simulink model "main"  (R2024a)
settings: Solver=FixedStepDiscrete  StartTime=0.0  StopTime=5  RelTol=1e-3
PreLoadFcn:
  | RTWConfigurationCB('preloadfcn', bdroot);
model workspace (MAT data in the model file):
  fault_count = 0
undefined symbols (not defined in the file or in its folder): Call, Function
libraries: canmsglib x15, c280xlib x13, c2837xDlib x9, c2802xlib x8, simulink x4, slpidlib x1
(part 2 of 2)

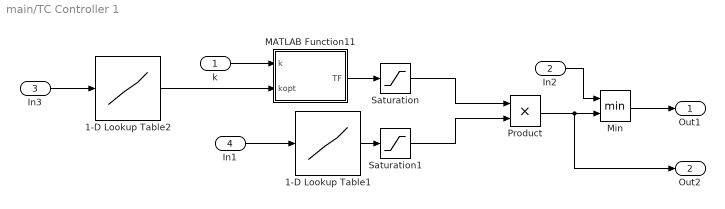
== system main/TC Controller 1 ==
  k : Inport
  In2 : Inport  Port=2
  In3 : Inport  Port=3
  In1 : Inport  Port=4
  1-D Lookup Table1 : Lookup_n-D  NumberOfTableDimensions=1  BreakpointsForDimension1=[1;10]  Table=[0;166]  ExtrapMethod=Clip  InternalRulePriority=Speed  RndMeth=Simplest
  1-D Lookup Table2 : Lookup_n-D  NumberOfTableDimensions=1  BreakpointsForDimension1=[1;10]  Table=[0.03;0.21]  ExtrapMethod=Clip  InternalRulePriority=Speed  RndMeth=Simplest
  MATLAB Function11 : MATLAB Function  TreatAsAtomicUnit=on
  Min : MinMax  Inputs=2
  Product : Product
  Saturation : Saturate  UpperLimit=1  LowerLimit=.1
  Saturation1 : Saturate  UpperLimit=166  LowerLimit=0
  Out1 : Outport
  Out2 : Outport  Port=2
  wires:
  1-D Lookup Table2/1 -> MATLAB Function11/2(kopt)
  MATLAB Function11/1(TF) -> Saturation/1
  Product/1 -> Out2/1, Min/2
  In1/1 -> 1-D Lookup Table1/1
  In2/1 -> Min/1
  1-D Lookup Table1/1 -> Saturation1/1
  Saturation1/1 -> Product/2
  Saturation/1 -> Product/1
  Min/1 -> Out1/1
  k/1 -> MATLAB Function11/1(k)
  In3/1 -> 1-D Lookup Table2/1

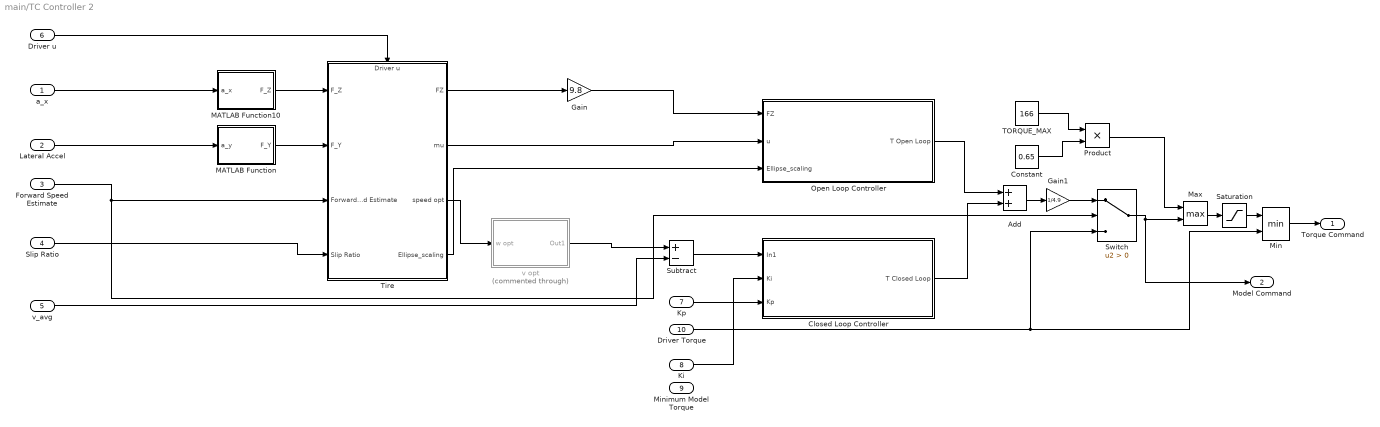
== system main/TC Controller 2 ==
  a_x : Inport
  Lateral Accel : Inport  Port=2
  Forward Speed Estimate : Inport  Port=3
  Slip Ratio : Inport  Port=4
  v_avg : Inport  Port=5
  Driver u : Inport  Port=6
  Kp : Inport  Port=7
  Ki : Inport  Port=8
  Minimum Model Torque : Inport  Port=9
  Driver Torque : Inport  Port=10
  Add : Sum
  Closed Loop Controller : Subsystem
  Constant : Constant  Value=0.65
  Gain : Gain  Gain=9.8
  Gain1 : Gain  Gain=1/4.9
  MATLAB Function : MATLAB Function  TreatAsAtomicUnit=on
  MATLAB Function10 : MATLAB Function  TreatAsAtomicUnit=on
  Max : MinMax  Function=max  Inputs=2
  Min : MinMax  Inputs=2
  Open Loop Controller : Subsystem
  Product : Product
  Saturation : Saturate  UpperLimit=166  LowerLimit=0
  Subtract : Sum  Inputs=+-
  Switch : Switch  Criteria=u2 > Threshold  SaturateOnIntegerOverflow=off  InputSameDT=off
  TORQUE_MAX : Constant  Value=166
  Tire : Subsystem
      settings: PortSchema="{\"entries\":[{\"content\":{\"sides\":[{\"content\":{\"connectorIds\":[\"In1\",\"In2\",\"In3\",\"In4\"]},\"type\":\"ConnectorPlacement.EquallySpacedRectSide\",\"uuid\":\"4156dcb8-571a-4ee4-a7f1-7560a1681aa7\"},{\"content\":{\"connectorIds\":[\"Out1\",\"Out2\",\"Out3\",\"Out4\"],\"side\":\"RIGHT\"},\"type\":\"ConnectorPlacement.EquallySpacedRectSide\",\"uuid\":\"73638d28-b906-4671-b83f-ad6b48e8d393\"},{\"content\":{\"connectorIds\":[\"In5\"],\"side\":\"TOP\"},\"type\":\"ConnectorPlacement.EquallySpacedRectSide\",\"uuid\":\"2e0ca522-3e79-4dd0-9128-59b05a2bd3de\"}]},\"type\":\"ConnectorPlacement.EquallySpacedConnector\",\"uuid\":\"62676716-b41d-4cd9-a12c-b09e0afde3e3\"}],\"packageUris\":[\"http://schema.mathworks.com/mf0/Connector/R2020b\"],\"version\":\"1.0\"}"
  v opt : Subsystem  Commented=through
  Torque Command : Outport
  Model Command : Outport  Port=2
  wires:
  Gain1/1 -> Switch/1
  Tire/2(mu) -> Open Loop Controller/2(u)
  a_x/1 -> MATLAB Function10/1(a_x)
  MATLAB Function10/1(F_Z) -> Tire/1(F_Z)
  Open Loop Controller/1(T Open Loop) -> Add/1
  Closed Loop Controller/1(T Closed Loop) -> Add/2
  v opt/1(Out1) -> Subtract/1
  Tire/3(speed opt) -> v opt/1(w opt)
  Subtract/1 -> Closed Loop Controller/1(In1)
  Add/1 -> Gain1/1
  Tire/1(FZ) -> Gain/1
  Driver u/1 -> Tire/5(Driver u)
  v_avg/1 -> Subtract/2
  Slip Ratio/1 -> Tire/4(Slip Ratio)
  Kp/1 -> Closed Loop Controller/3(Kp)
  Saturation/1 -> Min/1
  Gain/1 -> Open Loop Controller/1(FZ)
  Forward Speed Estimate/1 -> Switch/2, Tire/3(Forward Speed Estimate)
  Switch/1 -> Max/2, Model Command/1
  Driver Torque/1 -> Min/2, Switch/3
  Min/1 -> Torque Command/1
  Ki/1 -> Closed Loop Controller/2(Ki)
  Max/1 -> Saturation/1
  TORQUE_MAX/1 -> Product/1
  Constant/1 -> Product/2
  Product/1 -> Max/1
  MATLAB Function/1(F_Y) -> Tire/2(F_Y)
  Lateral Accel/1 -> MATLAB Function/1(a_y)
  Tire/4(Ellipse_scaling) -> Open Loop Controller/3(Ellipse_scaling)

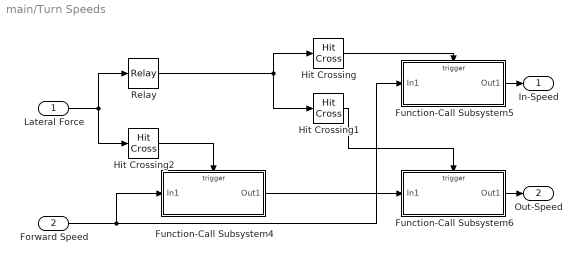
== system main/Turn Speeds ==
  Lateral Force : Inport
  Forward Speed : Inport  Port=2
  Function-Call Subsystem4 : Subsystem  TreatAsAtomicUnit=on
  Function-Call Subsystem5 : Subsystem  TreatAsAtomicUnit=on
  Function-Call Subsystem6 : Subsystem  TreatAsAtomicUnit=on
  Hit Crossing : HitCross  HitCrossingOffset=0.5  HitCrossingDirection=rising  HitCrossingOutputType=Function-Call
  Hit Crossing1 : HitCross  HitCrossingOffset=0.5  HitCrossingDirection=falling  HitCrossingOutputType=Function-Call
  Hit Crossing2 : HitCross  HitCrossingOffset=1  HitCrossingOutputType=Function-Call
  Relay : Relay  OnSwitchValue=1  OffSwitchValue=0.5
  In-Speed : Outport
  Out-Speed : Outport  Port=2
  wires:
  Forward Speed/1 -> Function-Call Subsystem4/1(In1), Function-Call Subsystem5/1(In1)
  Hit Crossing2/1 -> Function-Call Subsystem4/Trigger
  Function-Call Subsystem4/1(Out1) -> Function-Call Subsystem6/1(In1)
  Relay/1 -> Hit Crossing1/1, Hit Crossing/1
  Hit Crossing1/1 -> Function-Call Subsystem6/Trigger
  Hit Crossing/1 -> Function-Call Subsystem5/Trigger
  Function-Call Subsystem5/1(Out1) -> In-Speed/1
  Lateral Force/1 -> Relay/1, Hit Crossing2/1
  Function-Call Subsystem6/1(Out1) -> Out-Speed/1

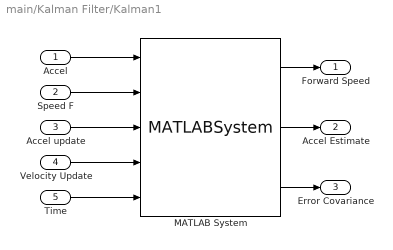
== system main/Kalman Filter/Kalman1 ==
  Accel : Inport
  Speed F : Inport  Port=2
  Accel update : Inport  Port=3
  Velocity Update : Inport  Port=4
  Time : Inport  Port=5
  MATLAB System : MATLABSystem  System=Kalman_Filter_Mod  qgain=1  SimulateUsing=Code generation
      mask Type: Kalman_Filter_Mod
      mask Display:
      | disp('Kalman_Filter_Mod');
      | port_label('input',1,'a');
      | port_label('input',2,'v_f');
      | port_label('input',3,'n_a');
      | port_label('input',4,'n_v');
      | port_label('input',5,'t_new');
      | port_label('output',1,'v');
      | port_label('output',2,'a');
      | port_label('output',3,'cov_v');
  Forward Speed : Outport
  Accel Estimate : Outport  Port=2
  Error Covariance : Outport  Port=3
  wires:
  Speed F/1 -> MATLAB System/2
  Accel/1 -> MATLAB System/1
  MATLAB System/1 -> Forward Speed/1
  Accel update/1 -> MATLAB System/3
  Velocity Update/1 -> MATLAB System/4
  Time/1 -> MATLAB System/5
  MATLAB System/2 -> Accel Estimate/1
  MATLAB System/3 -> Error Covariance/1

== system main/Kalman Filter/Sensor Driver 1 ==
  In1 : Inport
  Circumference : Gain  Gain=2*pi*0.203
  Gain : Gain  Gain=3.6
  Inverse Teeth : Gain  Gain=1/21
  " " : Outport
  wires:
  In1/1 -> Gain/1
  Gain/1 -> Circumference/1
  Circumference/1 -> Inverse Teeth/1
  Inverse Teeth/1 -> " "/1

== system main/Kalman Filter/Sensor Driver 2 ==
  In1 : Inport
  Circumference : Gain  Gain=2*pi*0.203
  Gain : Gain  Gain=3.6
  Inverse Teeth : Gain  Gain=1/21
  " " : Outport
  wires:
  Circumference/1 -> Inverse Teeth/1
  Inverse Teeth/1 -> " "/1
  In1/1 -> Gain/1
  Gain/1 -> Circumference/1

== system main/Kalman Filter/Sensor Driver 3 ==
  In1 : Inport
  Circumference : Gain  Gain=2*pi*0.203
  Gain : Gain  Gain=3.6
  Inverse Teeth : Gain  Gain=1/21
  RL : Outport
  wires:
  Circumference/1 -> Inverse Teeth/1
  Inverse Teeth/1 -> RL/1
  In1/1 -> Gain/1
  Gain/1 -> Circumference/1

== system main/Kalman Filter/Sensor Driver 4 ==
  In1 : Inport
  Circumference : Gain  Gain=2*pi*0.203
  Gain : Gain  Gain=3.6
  Inverse Teeth : Gain  Gain=1/21
  RR : Outport
  wires:
  Circumference/1 -> Inverse Teeth/1
  Inverse Teeth/1 -> RR/1
  In1/1 -> Gain/1
  Gain/1 -> Circumference/1

== system main/Kalman Filter/Slip Ratio Calculation1 ==
  RR : Inport
  Forward Speed : Inport  Port=2
  MATLAB Function : MATLAB Function  TreatAsAtomicUnit=on
  Slip Ratio : Outport
  wires:
  Forward Speed/1 -> MATLAB Function/1(fwd_speed)
  RR/1 -> MATLAB Function/2(v_rear)
  MATLAB Function/1(y) -> Slip Ratio/1

== system main/Power Limiting/Moving Average ==
  In1 : Inport
  Product1 : Product  Inputs=*/
  Saturation : Saturate  UpperLimit=inf  LowerLimit=1
  Sum of Elements : Sum  Inputs=+
  Tapped Delay : simulink/Discrete/Tapped Delay  vinit=0.0  samptime=-1  NumDelays=10  DelayOrder=Oldest  includeCurrent=on
  Width : Width
  Out1 : Outport
  wires:
  Tapped Delay/1 -> Width/1, Sum of Elements/1
  Sum of Elements/1 -> Product1/1
  Product1/1 -> Out1/1
  In1/1 -> Tapped Delay/1
  Width/1 -> Saturation/1
  Saturation/1 -> Product1/2

== system main/TC Controller 2/Closed Loop Controller ==
  In1 : Inport
  Ki : Inport  Port=2
  Kp : Inport  Port=3
  Constant : Constant  Value=2
  Divide : Product  Inputs=*/
  PID Controller : slpidlib/PID Controller  Controller=PI  Form=Parallel  TimeDomain=Discrete-time  UseExternalTs=off  SampleTime=-1  IntegratorMethod=Forward Euler  FilterMethod=Forward Euler  ControllerParametersSource=external  P=100  I=10  UseKiTs=off  D=0  UseExternalDerivativeSource=off  N=100  UseFilter=on  TunerSelectOption=Transfer Function Based (PID Tuner App)  InitialConditionSource=internal  InitialConditionForIntegrator=0  InitialConditionForFilter=0  DifferentiatorICPrevScaledInput=0  ExternalReset=none  TrackingMode=off  Kt=1  LimitOutput=on  SatLimitsSource=internal  UpperSaturationLimit=166  LowerSaturationLimit=0  LinearizeAsGain=on  AntiWindupMode=clamping  Kb=1  LimitIntegrator=on  UpperIntegratorSaturationLimit=166  LowerIntegratorSaturationLimit=0  POutMin=[]  POutMax=[]  IOutMin=[]  IOutMax=[]  DOutMin=[]  DOutMax=[]  NOutMin=[]  NOutMax=[]  SumOutMin=[]  SumOutMax=[]  SaturationOutMin=[]  SaturationOutMax=[]  PParamMin=[]  PParamMax=[]  IParamMin=[]  IParamMax=[]  DParamMin=[]  DParamMax=[]  NParamMin=[]  NParamMax=[]  KbParamMin=[]  KbParamMax=[]  KtParamMin=[]  KtParamMax=[]  KbOutMin=[]  KbOutMax=[]  KtOutMin=[]  KtOutMax=[]  IntegratorOutMin=[]  IntegratorOutMax=[]  FilterOutMin=[]  FilterOutMax=[]  SumI1OutMin=[]  SumI1OutMax=[]  SumI2OutMin=[]  SumI2OutMax=[]  SumI3OutMin=[]  SumI3OutMax=[]  SumI4OutMin=[]  SumI4OutMax=[]  SumDOutMin=[]  SumDOutMax=[]  DifferentiatorOutMin=[]  DifferentiatorOutMax=[]  FilterDiffOutCoefMin=[]  FilterDiffOutCoefMax=[]  ReciprocalOutMin=[]  ReciprocalOutMax=[]  SumDenOutMin=[]  SumDenOutMax=[]  SumNumOutMin=[]  SumNumOutMax=[]  DivideOutMin=[]  DivideOutMax=[]  UdiffTsProdOutMin=[]  UdiffTsProdOutMax=[]  NTsProdOutMin=[]  NTsProdOutMax=[]  UintegralTsProdOutMin=[]  UintegralTsProdOutMax=[]  UngainTsProdOutMin=[]  UngainTsProdOutMax=[]  ClampingZeroOutDataTypeStr=Inherit: Inherit via back propagation  ClampingZeroOutMin=[]  ClampingZeroOutMax=[]  FilterDenConstantOutDataTypeStr=Inherit: Inherit via back propagation  FilterDenConstantOutMin=[]  FilterDenConstantOutMax=[]  PCopyOutDataTypeStr=Inherit: Inherit via back propagation  PCopyOutMin=[]  PCopyOutMax=[]  NCopyOutDataTypeStr=Inherit: Inherit via back propagation  NCopyOutMin=[]  NCopyOutMax=[]  IntegratorContinuousStateAttributes=''  IntegratorStateMustResolveToSignalObject=off  IntegratorRTWStateStorageClass=Auto  FilterContinuousStateAttributes=''  FilterStateMustResolveToSignalObject=off  FilterRTWStateStorageClass=Auto  ParallelPVariant=ExternalParameters  IdealPVariant=Disabled  IVariant=ExternalParameters  DVariant=Disabled  IntegratorVariant=Discrete  SatVariant=Enabled  AWVariant=DiscClampingParallel  PCopyVariant=Disabled  TRVariant=Disabled  FdbkBlocksVariant=Forward  IdealPFdbkVariant=Disabled  SatFdbkVariant=Disabled  DerivativeFilterVariant=Disabled  NVariant=Disabled  NCopyVariant=Disabled_SignalSpec  FilterICVariant=Disabled  IntegratorICVariant=InternalICs  ExternalResetVariant=Disabled  TRSumVariant=Passthrough  SumFdbkVariant=Disabled  SumVariant=Sum_PI  TsampFilterVariant=InternalTs  TsampNgainVariant=Passthrough  TsampIntegralVariant=Disabled_SignalSpec  ExternalSaturationOutDataTypeStr=Inherit: Same as second input  DerivativeSourceVariant=Disabled
  T Closed Loop : Outport
  wires:
  In1/1 -> PID Controller/1
  PID Controller/1 -> T Closed Loop/1
  Kp/1 -> Divide/1, PID Controller/2
  Divide/1 -> ?
  Constant/1 -> Divide/2
  Ki/1 -> PID Controller/3

== system main/TC Controller 2/Open Loop Controller ==
  FZ : Inport
  u : Inport  Port=2
  Ellipse_scaling : Inport  Port=3
  Gain : Gain  Gain=0.203
  Product : Product
  Product1 : Product
  T Open Loop : Outport
  wires:
  FZ/1 -> Product/1
  u/1 -> Product/2
  Product/1 -> Product1/1
  Gain/1 -> T Open Loop/1
  Product1/1 -> Gain/1
  Ellipse_scaling/1 -> Product1/2

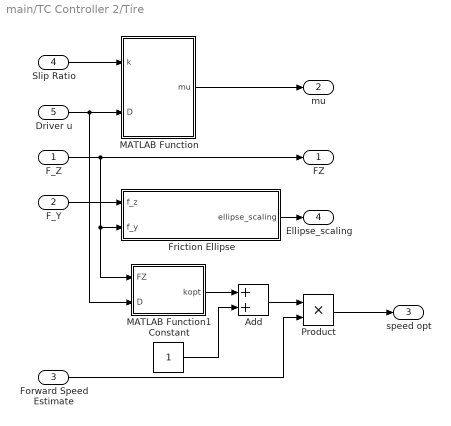
== system main/TC Controller 2/Tire ==
  F_Z : Inport
  F_Y : Inport  Port=2
  Forward Speed Estimate : Inport  Port=3
  Slip Ratio : Inport  Port=4
  Driver u : Inport  Port=5
  Add : Sum
  Constant : Constant
  Friction Ellipse : MATLAB Function  TreatAsAtomicUnit=on
  MATLAB Function : MATLAB Function  TreatAsAtomicUnit=on
  MATLAB Function1 : MATLAB Function  TreatAsAtomicUnit=on
  Product : Product
  FZ : Outport
  mu : Outport  Port=2
  speed opt : Outport  Port=3
  Ellipse_scaling : Outport  Port=4
  wires:
  F_Z/1 -> FZ/1, Friction Ellipse/2(f_y), MATLAB Function1/1(FZ)
  Driver u/1 -> MATLAB Function/2(D), MATLAB Function1/2(D)
  Slip Ratio/1 -> MATLAB Function/1(k)
  MATLAB Function/1(mu) -> mu/1
  Constant/1 -> Add/2
  MATLAB Function1/1(kopt) -> Add/1
  Add/1 -> Product/1
  Forward Speed Estimate/1 -> Product/2
  Product/1 -> speed opt/1
  F_Y/1 -> Friction Ellipse/1(f_z)
  Friction Ellipse/1(ellipse_scaling) -> Ellipse_scaling/1

== system main/TC Controller 2/v opt ==
  w opt : Inport
  Circumference : Gain  Gain=2*pi*0.203
  Gain1 : Gain  Gain=3.6
  Out1 : Outport
  wires:
  Circumference/1 -> Out1/1
  w opt/1 -> Gain1/1
  Gain1/1 -> Circumference/1

== system main/Turn Speeds/Function-Call Subsystem4 ==
  In1 : Inport
  function : TriggerPort  TriggerType=function-call  VariantControl=(inherit)
  Out1 : Outport
  wires:
  In1/1 -> Out1/1

== system main/Turn Speeds/Function-Call Subsystem5 ==
  In1 : Inport
  function : TriggerPort  TriggerType=function-call  VariantControl=(inherit)
  Out1 : Outport
  wires:
  In1/1 -> Out1/1

== system main/Turn Speeds/Function-Call Subsystem6 ==
  In1 : Inport
  function : TriggerPort  TriggerType=function-call  VariantControl=(inherit)
  Out1 : Outport
  wires:
  In1/1 -> Out1/1

== matlab function main/MATLAB Function ==
  data: ts input; out output int8; length input
function out = fcn(ts, length)

% if timeout
%     out = -1; % timeout in TS state CAN signal
persistent timeout;
if isempty(timeout)
    timeout = 0;
end

if length == 0
    timeout = timeout + 1;
else
    timeout = 0;
end

if timeout > 4
    out = int8(-1);
else
    out = int8(ts);
end

== stateflow chart main/Chart ==
  state State6_Motor_Disabled
    state=6;
    ready_led = 0;
    buzzer = 0;
    inverter_en = 0;
    dc_dc = 1;
    driving = 0;
  state State1_TS_NotReady
    state=1;
    ready_led = 0;
    buzzer = 0;
    inverter_en = 0;
    dc_dc = 0;
    driving = 0;
  state State5_Ready_to_Drive
    state=5;
    ready_led = 0;
    buzzer = 0;
    inverter_en = 1;
    dc_dc = 1;
    driving = 1;
  state State4_Enabling
    state=4;
    ready_led = 0;
    buzzer = 0;
    inverter_en = 1;
    dc_dc = 1;
    driving = 0;
  state State3_Buzzing
    state=3;
    ready_led = 0;
    buzzer = 1;
    inverter_en = 0;
    dc_dc = 1;
    driving = 0;
  state State2_TS_Ready
    state=2;
    ready_led = 1;
    buzzer = 0;
    inverter_en = 0;
    dc_dc = 0;
    driving = 0;
  State3_Buzzing -> State1_TS_NotReady [order 2] : [TS_state ~= 3]
  State5_Ready_to_Drive -> State1_TS_NotReady [order 2] : [TS_state ~= 3]
  State6_Motor_Disabled -> State1_TS_NotReady [order 1] : [TS_state ~= 3]
  (default) -> State1_TS_NotReady
  State4_Enabling -> State6_Motor_Disabled [order 2] : [any(Pedal_Fault)]
  State6_Motor_Disabled -> State4_Enabling [order 2] : [~any(Pedal_Fault)]
  State5_Ready_to_Drive -> State6_Motor_Disabled [order 1] : [any(Pedal_Fault)]
  State2_TS_Ready -> State1_TS_NotReady [order 2] : [TS_state ~= 3]
  State1_TS_NotReady -> State2_TS_Ready : [TS_state == 3]
  State5_Ready_to_Drive -> State2_TS_Ready [order 3] : [INV_enable ~= 1]
  State4_Enabling -> State5_Ready_to_Drive [order 1] : [INV_enable==1]
  State3_Buzzing -> State4_Enabling [order 1] : after(3,sec)
  State2_TS_Ready -> State3_Buzzing [order 1] : [BPT==1&&RTD_Button==1]
  data: BPT input; RTD_Button input; Pedal_Fault input; INV_enable input; TS_state input; state output; ready_led output; buzzer output; dc_dc output; inverter_en output; driving output

== matlab function main/MATLAB Function2 ==
  data: can_ok input; timeout output
function timeout = ts_chilin(can_ok)

persistent counter;
TS_CAN_COUNT = 3; % 3 samples at 10Hz is a 300ms timeout

% initialize counter
if isempty(counter)
    counter = 0;
end

if can_ok
    counter = 0;
else
    counter = counter + 1;
end

if counter > TS_CAN_COUNT
    timeout = 1;
else
    timeout = 0;
end

== matlab function main/MATLAB Function3 ==
  data: inv input; out output int8; length input
function out = fcn(inv, length)

% if timeout
%     out = -1; % timeout in TS state CAN signal
persistent timeout;
if isempty(timeout)
    timeout = 0;
end

if length == 0
    timeout = timeout + 1;
else
    timeout = 0;
end

if timeout > 4
    out = int8(-1);
else
    out = int8(inv);
end

== matlab function main/MATLAB Function4 ==
  data: sig input; APPS1_RANGE input; r_momentary input; percent output
function percent = map_apps1(sig, APPS1_RANGE, r_momentary)

DZ_BOT = .05; %rosnel changed to .05 was .1 
DZ_TOP = .05; 

APPS_BOTTOM = APPS1_RANGE(1) + DZ_BOT * (APPS1_RANGE(2) - APPS1_RANGE(1)) ;
APPS_TOP    = APPS1_RANGE(2) - DZ_TOP * (APPS1_RANGE(2) - APPS1_RANGE(1)) ;

if (sig < APPS_BOTTOM) || r_momentary(1) || r_momentary(2)
    percent = 0;
elseif sig > APPS_TOP
    percent = 1;
else
    percent = (double(sig) - APPS_BOTTOM) / (APPS_TOP - APPS_BOTTOM);
end

== matlab function main/MATLAB Function5 ==
  data: can_ok input; timeout output
function timeout = inv_chillin(can_ok)

persistent counter;
INV_CAN_COUNT = 3; % 3 samples at 10Hz is a 300ms timeout

% initialize counter
if isempty(counter)
    counter = 0;
end

if can_ok
    counter = 0;
else
    counter = counter + 1;
end

if counter > INV_CAN_COUNT
    timeout = 1;
else
    timeout = 0;
end

== matlab function main/MATLAB Function6 ==
  data: ped input; torque output; knob input; TORQUE_MAX input
function torque = fcn(ped, knob, TORQUE_MAX)

t = ped * knob;
torque = min(max(t, 0), 1);

torque = t * TORQUE_MAX;

== matlab function main/MATLAB Function7 ==
  data: driving input; pedal_torque input; direction output; discharge output; enable output; counter output; speed output; speed_mode output; torque output; torque_limit output
function [direction, discharge, enable, counter, speed, speed_mode, torque, torque_limit]   = fcn(driving, pedal_torque)

persistent my_counter;
if isempty(my_counter)
    my_counter = 0;
else
    my_counter = mod(my_counter + 1, 16);
end

counter = my_counter;

if driving == 1
    torque = pedal_torque;
    speed = 0;
    direction = 1;
    enable = 1;
    discharge = 0;
    speed_mode = 0;
    torque_limit = 0;
else
    torque = 0;
    speed = 0;
    direction = 0;
    enable = 0;
    discharge = 0;
    speed_mode = 0;
    torque_limit = 0;
end

== matlab function main/Kalman Filter/MATLAB Function6 ==
  data: v_rl input; v_rear output; v_rr input
function v_rear = fcn(v_rl,v_rr)
if(v_rl == 0)
    v_rear = v_rr;
elseif(v_rr == 0)
    v_rear = v_rl;
else
    v_rear= (v_rl+v_rr)/2;
end
end

== matlab function main/MATLAB Function9 ==
  data: r_fault_counts output; r_faults output; bpt_sig_mcu input; apps_sig1_mcu input; apps_sig2_mcu input; APPS1_OP input; APPS2_OP input; BPTF_ENGAGED input; APPS1_FAULT input; APPS2_FAULT input; BPTF_FAULT input; r_momentary output
function [r_fault_counts, r_faults, r_momentary] = fcn(bpt_sig_mcu, apps_sig1_mcu, apps_sig2_mcu, APPS1_OP, APPS2_OP, BPTF_ENGAGED, APPS1_FAULT, APPS2_FAULT, BPTF_FAULT)
%#codegen
%To map voltages / integers:
%Pre step down voltages (from sensors, range 0 to 5 V) * 2/3 -> Post step down voltages (0 to 3.3 V, used by mcu)
%Post step down voltages * (4096 / 3.3) -> uint16 (integer) value of variables
%Note: Some values are tweaked after testing to handle noise. 455 -> 435, 0.1 -> 0.13, etc. All values can and should be optimized from testing, especially from testing on the car

%Current operating range (MCU): 0.32 V to 2.67 V
%Brakes considered pressed: 0.40 V
%typical MCU noise: +- 0.03V

persistent fault_counts;
persistent faults;

FAULT_LIMITS = [10, 10, 10, 10, 10, 10, 10, 1];

% initialize persistents
if isempty(fault_counts)
    fault_counts = zeros(1,8);
end

if isempty(faults)
    faults = [false, false, false, false, false, false, false, false];
end

apps1_percent_pressed = (double(apps_sig1_mcu) - APPS1_OP(1))/(APPS1_OP(2) - APPS1_OP(1)); % current travel divided by range of travel
apps2_percent_pressed = (double(apps_sig2_mcu) - APPS2_OP(1))/(APPS2_OP(2) - APPS2_OP(1));

% Clear fault case 8 (two pedals) when apps goes below 5% travel
if (apps1_percent_pressed < 0.05)
    faults(8) = 0;
    fault_counts(8) = 0;
end

% Cases 1-6: APPS or BPT out of operating range (sensor failure)
out_of_bounds = [apps_sig1_mcu < APPS1_FAULT(1), apps_sig1_mcu > APPS1_FAULT(2), ...
                 apps_sig2_mcu < APPS2_FAULT(1), apps_sig2_mcu > APPS2_FAULT(2), ...
                 bpt_sig_mcu   < BPTF_FAULT(1),  bpt_sig_mcu   > BPTF_FAULT(2)];
% Case 7: Both APPS sensors differ by more than 10% for more than 100ms. 
apps_disagree = abs(apps1_percent_pressed - apps2_percent_pressed) > 0.1;
% Case 8: If APPS is more than 25% pressed and brakes are pressed.
two_pedal = (apps1_percent_pressed >= 0.25) && (bpt_sig_mcu >= BPTF_ENGAGED);

conditions = [out_of_bounds, apps_disagree, two_pedal];

r_momentary = conditions;

conditions(8) = conditions(8) || faults(8); % Case 8 is sticky

% if condition is met but haven't yet triggered fault, increment fault_count.
% if condition is met but already in fault, leave fault_count the same (to
% prevent overflow)
% if condition is not met, zero the count
fault_counts = conditions .* (fault_counts + not(faults));
faults = fault_counts >= FAULT_LIMITS;

r_fault_counts = fault_counts;
r_faults = faults;

== matlab function main/Kalman Filter/MATLAB Function8 ==
  data: v_fl input; v_front output; v_fr input
function v_front = fcn(v_fl,v_fr)

if(v_fl == 0)
    v_front = v_fr;
elseif(v_fr == 0)
    v_front = v_fl;
else
    v_front= (v_fl+v_fr)/2;
end
end

== matlab function main/Kalman Filter/Slip Ratio Calculation1/MATLAB Function ==
  data: fwd_speed input; y output; v_rear input
function y = fcn(fwd_speed,v_rear)

y = (v_rear - fwd_speed)/(max([fwd_speed,0.1]));

== matlab function main/TC Controller 2/MATLAB Function ==
  data: a_y input; F_Y output
function F_Y = fcn(a_y)
m = 250+68; %Mass with driver weight
a = 1.530/2; %Distance cg to front axle with load distribution of 0.5
h = 0.249; %Height of CG
l = 1.530; %Length of wheelbase
F_Y = (a/l)*m*a_y;

== matlab function main/Motec Screen/MATLAB Function10 ==
  data: l input; page output; r input
function page = fcn(l,r)

persistent m_page;
if isempty(m_page)
    m_page = 0;
end

if(l~=0)
    if (m_page > 0)
        m_page=m_page-1;
    end
elseif(r~=0)
    if (m_page < 4)
        m_page=m_page+1;
    end
end

page = m_page;

== matlab function main/TC Controller 2/MATLAB Function10 ==
  data: a_x input; F_Z output
function F_Z = fcn(a_x)
m = 250+68; %Mass with driver weight
a = 1.530/2; %Distance cg to front axle with load distribution of 0.5
h = 0.249; %Height of CG
l = 1.530; %Length of wheelbase
F_Z = m*(2*a+h*a_x)/(2*l);

== matlab function main/TC Controller 2/Tire/MATLAB Function ==
  data: k input; mu output; D input
function mu = fcn(k,D)
C=1.5926; % [1]
B=11.8721; % [1]
E=0;
mu = D*sin(C*atan(B*k-E*(B*k-atan(B*k))));

== matlab function main/TC Controller 2/Tire/MATLAB Function1 ==
  data: FZ input; D input; kopt output
function kopt = fcn(FZ, D)
% something blah differential this(B - E*(B - B/(B^2*k^2 + 1)))/((B*k + E*(atan(B*k) - B*k))^2 + 1)

B = 7.9557; C = 1.9778; D = 2142.5492; E = 0.3682;

persistent k;
if isempty(k)
    k = 0;
end

if k < 0
    k = 0;
end

T = sin(C*atan(B*k-E*(B*k-atan(B*k))));
dT_dk = (C*cos(C*atan(B*k + E*(atan(B*k) - B*k)))*(B - E*(B - B/(B^2*k^2 + 1))))/((B*k + E*(atan(B*k) - B*k))^2 + 1);

if abs(dT_dk) > 0.05
    k = k + 0.01 * dT_dk;
end


kopt = k;

== matlab function main/TC Controller 2/Tire/Friction Ellipse ==
  data: f_z input; f_y input; ellipse_scaling output
function ellipse_scaling = fcn(f_z, f_y)
u_ymax = 1.36;
ellipse_scaling = sqrt(1-(f_y/(u_ymax*f_z))^2);

== matlab function main/TC Controller 1/MATLAB Function11 ==
  data: k input; TF output; kopt input
function TF = fcn(k, kopt)
r=.025;
if (k < kopt-r)
    TF = 1-(kopt-r-k)*0.8;
elseif (k > kopt+r)
    TF = 1-(k-kopt-r)*1.2;
else
    TF = 1;
end

== matlab function main/MATLAB Function10 ==
  data: u input; y output
function y = fcn(u)
if u==1 || u==2 
    y = 1;
else
    y = 0;
end

== matlab function main/Pedals Curve Switcher/MATLAB Function ==
  data: exp input; table output
function table = fcn(exp)
table = linspace(0,1,100).^exp;

== matlab function main/MATLAB Function1 ==
  data: u input; y output; time input
function y = fcn(u,time)
persistent curr_time;
persistent flag;
if isempty(curr_time)
    curr_time = 0;
end
if isempty(flag)
    flag = 0;
end
if u && time > 10
    curr_time = time;
    flag = 1;
end
if time < (curr_time+35) && flag
y = 1;
else 
y=0;
flag = 0;
end
